simulink library "halin"  (R2021b)
settings: Solver=VariableStepAuto  StartTime=0.0  StopTime=10.0  RelTol=1e-3
undefined symbols (not defined in the file): KHAL_CAN1ABM1E2E_flg, KHAL_CAN1ESC1E2E_flg, KHAL_CAN1ESC5E2E_flg, KHAL_CAN1ESC7E2E_flg, KHAL_CAN1FCM2E2E_flg, KHAL_CAN1FCM3E2E_flg, KHAL_CAN1FCM4E2E_flg, KHAL_CAN3BMS1E2E_flg, KHAL_CAN3BMS6E2E_flg, KHAL_CAN3CCU1E2E_flg, KHAL_CAN3CCU2E2E_flg, KHAL_CAN3MCUF1E2E_flg, KHAL_CAN3MCUR1E2E_flg, KHAL_CAN3Shifter1E2E_flg, TRUE
libraries: simulink x420, FVT_lib x149, hcu_lib x49
(part 2 of 14)

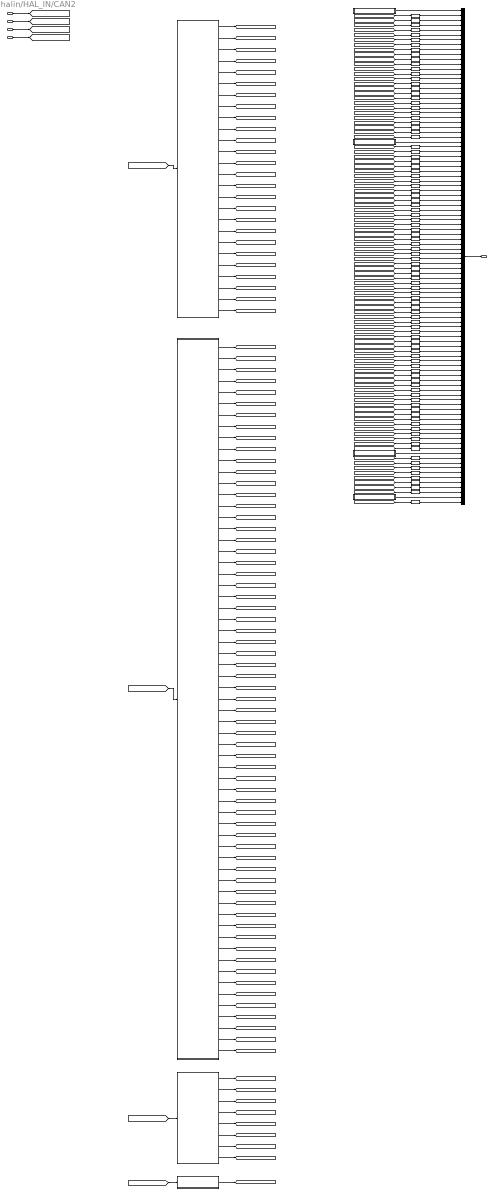
== system halin/HAL_IN/CAN2 ==
  DT_CAN2_SG_IVI1 : Inport
  DT_CAN2_SG_IVI2 : Inport  Port=2
  DT_CAN2_SG_IVI6 : Inport  Port=3
  DT_CAN2_SG_METER1 : Inport  Port=4
  IVI1 : Subsystem
  IVI2 : Subsystem
  IVI6 : Subsystem
  METER1 : Subsystem
  UnitConverter{,1,11,25,28..30,32,37..39,43..44,46,48..50,52..53,57,66..68,70,75,77,80,82,89..90} (30 alike) : DataTypeConversion  OutDataTypeStr=uint8
  UnitConverter{2,4..8,10,12..24,26..27,31,33..36,40,45,47,51,54..56,58..60,69,71,73..74,76,78..79,81,83..86} (49 alike) : DataTypeConversion  OutDataTypeStr=boolean
  UnitConverter{3,9,41,61..65,72,87..88,91..97} (18 alike) : DataTypeConversion  OutDataTypeStr=single
  UnitConverter42 : DataTypeConversion  OutDataTypeStr=uint32
  VHAL_CANMsgInvalidIVI1_flg : Subsystem  AncestorBlock=FVT_lib/hal/MsgTimeoutJudge_CAN_AUTOSAR
      mask help: MeasumentTrigerEvent
      mask Display: fprintf('MsgTimeoutJudge_CAN\nAUTOSAR');
  VHAL_CANMsgInvalidIVI2_flg : Subsystem  AncestorBlock=FVT_lib/hal/MsgTimeoutJudge_CAN_AUTOSAR
      mask help: MeasumentTrigerEvent
      mask Display: fprintf('MsgTimeoutJudge_CAN\nAUTOSAR');
  VHAL_CANMsgInvalidIVI6_flg : Subsystem  AncestorBlock=FVT_lib/hal/MsgTimeoutJudge_CAN_AUTOSAR
      mask help: MeasumentTrigerEvent
      mask Display: fprintf('MsgTimeoutJudge_CAN\nAUTOSAR');
  VHAL_CANMsgInvalidMETER1_flg : Subsystem  AncestorBlock=FVT_lib/hal/MsgTimeoutJudge_CAN_AUTOSAR
      mask help: MeasumentTrigerEvent
      mask Display: fprintf('MsgTimeoutJudge_CAN\nAUTOSAR');
  bus_creator : BusCreator  Inputs=102
  HAL_CAN2_outputs : Outport
  wires:
  DT_CAN2_SG_IVI1/1 -> [DT_CAN2_SG_IVI1]
  DT_CAN2_SG_IVI2/1 -> [DT_CAN2_SG_IVI2]
  DT_CAN2_SG_IVI6/1 -> [DT_CAN2_SG_IVI6]
  DT_CAN2_SG_METER1/1 -> [DT_CAN2_SG_METER1]
  [DT_CAN2_SG_IVI1] -> IVI1/1(DT_CAN2_SG_IVI1)
  [DT_CAN2_SG_IVI2] -> IVI2/1(DT_CAN2_SG_IVI2)
  [DT_CAN2_SG_IVI6] -> IVI6/1(DT_CAN2_SG_IVI6)
  [DT_CAN2_SG_METER1] -> METER1/1(DT_CAN2_SG_METER1)
  bus_creator/1 -> HAL_CAN2_outputs/1
  VHAL_CANMsgInvalidIVI1_flg/1(Out) -> bus_creator/1
  IVI1/1(VHAL_AmbLightColorSet_enum) -> [VHAL_AmbLightColorSet_enum]
  UnitConverter/1 -> bus_creator/2  "VHAL_AmbLightColorSet_enum"
  [VHAL_AmbLightColorSet_enum] -> UnitConverter/1
  IVI1/2(VHAL_AmbLightUserSet_enum) -> [VHAL_AmbLightUserSet_enum]
  UnitConverter1/1 -> bus_creator/3  "VHAL_AmbLightUserSet_enum"
  [VHAL_AmbLightUserSet_enum] -> UnitConverter1/1
  IVI1/3(VHAL_BrkAbnGoReadySW_flg) -> [VHAL_BrkAbnGoReadySW_flg]
  UnitConverter2/1 -> bus_creator/4  "VHAL_BrkAbnGoReadySW_flg"
  [VHAL_BrkAbnGoReadySW_flg] -> UnitConverter2/1
  IVI1/4(VHAL_DRAmbLightBrightnessSet_pct) -> [VHAL_DRAmbLightBrightnessSet_pct]
  UnitConverter3/1 -> bus_creator/5  "VHAL_DRAmbLightBrightnessSet_pct"
  [VHAL_DRAmbLightBrightnessSet_pct] -> UnitConverter3/1
  IVI1/5(VHAL_FCPFrEvtBtnACMaxReq_flg) -> [VHAL_FCPFrEvtBtnACMaxReq_flg]
  UnitConverter4/1 -> bus_creator/6  "VHAL_FCPFrEvtBtnACMaxReq_flg"
  [VHAL_FCPFrEvtBtnACMaxReq_flg] -> UnitConverter4/1
  IVI1/6(VHAL_FCPFrEvtBtnACReq_flg) -> [VHAL_FCPFrEvtBtnACReq_flg]
  UnitConverter5/1 -> bus_creator/7  "VHAL_FCPFrEvtBtnACReq_flg"
  [VHAL_FCPFrEvtBtnACReq_flg] -> UnitConverter5/1
  IVI1/7(VHAL_FCPFrEvtBtnAutoReq_flg) -> [VHAL_FCPFrEvtBtnAutoReq_flg]
  UnitConverter6/1 -> bus_creator/8  "VHAL_FCPFrEvtBtnAutoReq_flg"
  [VHAL_FCPFrEvtBtnAutoReq_flg] -> UnitConverter6/1
  IVI1/8(VHAL_FCPFrEvtBtnSyncReq_flg) -> [VHAL_FCPFrEvtBtnSyncReq_flg]
  UnitConverter7/1 -> bus_creator/9  "VHAL_FCPFrEvtBtnSyncReq_flg"
  [VHAL_FCPFrEvtBtnSyncReq_flg] -> UnitConverter7/1
  IVI1/9(VHAL_FCPMidEvtBtnAutoReq_flg) -> [VHAL_FCPMidEvtBtnAutoReq_flg]
  UnitConverter8/1 -> bus_creator/10  "VHAL_FCPMidEvtBtnAutoReq_flg"
  [VHAL_FCPMidEvtBtnAutoReq_flg] -> UnitConverter8/1
  IVI1/10(VHAL_IPAmbLightBrightnessSet_pct) -> [VHAL_IPAmbLightBrightnessSet_pct]
  UnitConverter9/1 -> bus_creator/11  "VHAL_IPAmbLightBrightnessSet_pct"
  [VHAL_IPAmbLightBrightnessSet_pct] -> UnitConverter9/1
  IVI1/11(VHAL_IVILockSoundSWSta_flg) -> [VHAL_IVILockSoundSWSta_flg]
  UnitConverter10/1 -> bus_creator/12  "VHAL_IVILockSoundSWSta_flg"
  [VHAL_IVILockSoundSWSta_flg] -> UnitConverter10/1
  IVI1/12(VHAL_IVIOTAUpdSta_enum) -> [VHAL_IVIOTAUpdSta_enum]
  UnitConverter11/1 -> bus_creator/13  "VHAL_IVIOTAUpdSta_enum"
  [VHAL_IVIOTAUpdSta_enum] -> UnitConverter11/1
  IVI1/13(VHAL_LINKtoDrive_flg) -> [VHAL_LINKtoDrive_flg]
  UnitConverter12/1 -> bus_creator/14  "VHAL_LINKtoDrive_flg"
  [VHAL_LINKtoDrive_flg] -> UnitConverter12/1
  IVI1/14(VHAL_OTACancelDLReq_flg) -> [VHAL_OTACancelDLReq_flg]
  UnitConverter13/1 -> bus_creator/15  "VHAL_OTACancelDLReq_flg"
  [VHAL_OTACancelDLReq_flg] -> UnitConverter13/1
  IVI1/15(VHAL_OTACompNTFYPres_flg) -> [VHAL_OTACompNTFYPres_flg]
  UnitConverter14/1 -> bus_creator/16  "VHAL_OTACompNTFYPres_flg"
  [VHAL_OTACompNTFYPres_flg] -> UnitConverter14/1
  IVI1/16(VHAL_OTADLReq_flg) -> [VHAL_OTADLReq_flg]
  UnitConverter15/1 -> bus_creator/17  "VHAL_OTADLReq_flg"
  [VHAL_OTADLReq_flg] -> UnitConverter15/1
  IVI1/17(VHAL_OTASuspendDLReq_flg) -> [VHAL_OTASuspendDLReq_flg]
  UnitConverter16/1 -> bus_creator/18  "VHAL_OTASuspendDLReq_flg"
  [VHAL_OTASuspendDLReq_flg] -> UnitConverter16/1
  IVI1/18(VHAL_OTAUpdStartReq_flg) -> [VHAL_OTAUpdStartReq_flg]
  UnitConverter17/1 -> bus_creator/19  "VHAL_OTAUpdStartReq_flg"
  [VHAL_OTAUpdStartReq_flg] -> UnitConverter17/1
  IVI1/19(VHAL_OpenDrOpenWdoSW_flg) -> [VHAL_OpenDrOpenWdoSW_flg]
  UnitConverter18/1 -> bus_creator/20  "VHAL_OpenDrOpenWdoSW_flg"
  [VHAL_OpenDrOpenWdoSW_flg] -> UnitConverter18/1
  IVI1/20(VHAL_PWCLOSEIMD_flg) -> [VHAL_PWCLOSEIMD_flg]
  UnitConverter19/1 -> bus_creator/21  "VHAL_PWCLOSEIMD_flg"
  [VHAL_PWCLOSEIMD_flg] -> UnitConverter19/1
  IVI1/21(VHAL_PWCONTINUEUSE_flg) -> [VHAL_PWCONTINUEUSE_flg]
  UnitConverter20/1 -> bus_creator/22  "VHAL_PWCONTINUEUSE_flg"
  [VHAL_PWCONTINUEUSE_flg] -> UnitConverter20/1
  IVI1/22(VHAL_SchedOTAwake_flg) -> [VHAL_SchedOTAwake_flg]
  UnitConverter21/1 -> bus_creator/23  "VHAL_SchedOTAwake_flg"
  [VHAL_SchedOTAwake_flg] -> UnitConverter21/1
  IVI1/23(VHAL_SmartEcoModeSW_flg) -> [VHAL_SmartEcoModeSW_flg]
  UnitConverter22/1 -> bus_creator/24  "VHAL_SmartEcoModeSW_flg"
  [VHAL_SmartEcoModeSW_flg] -> UnitConverter22/1
  IVI1/24(VHAL_UpdCountdownCancel_flg) -> [VHAL_UpdCountdownCancel_flg]
  UnitConverter23/1 -> bus_creator/25  "VHAL_UpdCountdownCancel_flg"
  [VHAL_UpdCountdownCancel_flg] -> UnitConverter23/1
  IVI1/25(VHAL_UpdCountdownSkip_flg) -> [VHAL_UpdCountdownSkip_flg]
  UnitConverter24/1 -> bus_creator/26  "VHAL_UpdCountdownSkip_flg"
  [VHAL_UpdCountdownSkip_flg] -> UnitConverter24/1
  IVI1/26(VHAL_VehACModReq_enum) -> [VHAL_VehACModReq_enum]
  UnitConverter25/1 -> bus_creator/27  "VHAL_VehACModReq_enum"
  [VHAL_VehACModReq_enum] -> UnitConverter25/1
  VHAL_CANMsgInvalidIVI2_flg/1(Out) -> bus_creator/28
  IVI2/1(VHAL_AVMErrSTA_flg) -> [VHAL_AVMErrSTA_flg]
  UnitConverter26/1 -> bus_creator/29  "VHAL_AVMErrSTA_flg"
  [VHAL_AVMErrSTA_flg] -> UnitConverter26/1
  IVI2/2(VHAL_AVMOFFRecButt_flg) -> [VHAL_AVMOFFRecButt_flg]
  UnitConverter27/1 -> bus_creator/30  "VHAL_AVMOFFRecButt_flg"
  [VHAL_AVMOFFRecButt_flg] -> UnitConverter27/1
  IVI2/3(VHAL_AVMParkingmode_enum) -> [VHAL_AVMParkingmode_enum]
  UnitConverter28/1 -> bus_creator/31  "VHAL_AVMParkingmode_enum"
  [VHAL_AVMParkingmode_enum] -> UnitConverter28/1
  IVI2/4(VHAL_AVMparkingcancel_enum) -> [VHAL_AVMparkingcancel_enum]
  UnitConverter29/1 -> bus_creator/32  "VHAL_AVMparkingcancel_enum"
  [VHAL_AVMparkingcancel_enum] -> UnitConverter29/1
  IVI2/5(VHAL_AVMparkingexcute_enum) -> [VHAL_AVMparkingexcute_enum]
  UnitConverter30/1 -> bus_creator/33  "VHAL_AVMparkingexcute_enum"
  [VHAL_AVMparkingexcute_enum] -> UnitConverter30/1
  IVI2/6(VHAL_ApproachUnlockSW_flg) -> [VHAL_ApproachUnlockSW_flg]
  UnitConverter31/1 -> bus_creator/34  "VHAL_ApproachUnlockSW_flg"
  [VHAL_ApproachUnlockSW_flg] -> UnitConverter31/1
  IVI2/7(VHAL_CAASSw_enum) -> [VHAL_CAASSw_enum]
  UnitConverter32/1 -> bus_creator/35  "VHAL_CAASSw_enum"
  [VHAL_CAASSw_enum] -> UnitConverter32/1
  IVI2/8(VHAL_CDLLockButt_flg) -> [VHAL_CDLLockButt_flg]
  UnitConverter33/1 -> bus_creator/36  "VHAL_CDLLockButt_flg"
  [VHAL_CDLLockButt_flg] -> UnitConverter33/1
  IVI2/9(VHAL_CDLUnlockButt_flg) -> [VHAL_CDLUnlockButt_flg]
  UnitConverter34/1 -> bus_creator/37  "VHAL_CDLUnlockButt_flg"
  [VHAL_CDLUnlockButt_flg] -> UnitConverter34/1
  IVI2/10(VHAL_DSEATantiset_flg) -> [VHAL_DSEATantiset_flg]
  UnitConverter35/1 -> bus_creator/38  "VHAL_DSEATantiset_flg"
  [VHAL_DSEATantiset_flg] -> UnitConverter35/1
  IVI2/11(VHAL_DSEATentryfunset_flg) -> [VHAL_DSEATentryfunset_flg]
  UnitConverter36/1 -> bus_creator/39  "VHAL_DSEATentryfunset_flg"
  [VHAL_DSEATentryfunset_flg] -> UnitConverter36/1
  IVI2/12(VHAL_DSEATventreq_enum) -> [VHAL_DSEATventreq_enum]
  UnitConverter37/1 -> bus_creator/40  "VHAL_DSEATventreq_enum"
  [VHAL_DSEATventreq_enum] -> UnitConverter37/1
  IVI2/13(VHAL_ESCSWCmd_enum) -> [VHAL_ESCSWCmd_enum]
  UnitConverter38/1 -> bus_creator/41  "VHAL_ESCSWCmd_enum"
  [VHAL_ESCSWCmd_enum] -> UnitConverter38/1
  IVI2/14(VHAL_FSOffSw_enum) -> [VHAL_FSOffSw_enum]
  UnitConverter39/1 -> bus_creator/42  "VHAL_FSOffSw_enum"
  [VHAL_FSOffSw_enum] -> UnitConverter39/1
  IVI2/15(VHAL_FollowMeSW_flg) -> [VHAL_FollowMeSW_flg]
  UnitConverter40/1 -> bus_creator/43  "VHAL_FollowMeSW_flg"
  [VHAL_FollowMeSW_flg] -> UnitConverter40/1
  IVI2/16(VHAL_GPSLAT_s) -> [VHAL_GPSLAT_s]
  UnitConverter41/1 -> bus_creator/44  "VHAL_GPSLAT_s"
  [VHAL_GPSLAT_s] -> UnitConverter41/1
  IVI2/17(VHAL_GPSLONG_enum) -> [VHAL_GPSLONG_enum]
  UnitConverter42/1 -> bus_creator/45  "VHAL_GPSLONG_enum"
  [VHAL_GPSLONG_enum] -> UnitConverter42/1
  IVI2/18(VHAL_HeadLampSW_enum) -> [VHAL_HeadLampSW_enum]
  UnitConverter43/1 -> bus_creator/46  "VHAL_HeadLampSW_enum"
  [VHAL_HeadLampSW_enum] -> UnitConverter43/1
  IVI2/19(VHAL_HoodLatchSW_enum) -> [VHAL_HoodLatchSW_enum]
  UnitConverter44/1 -> bus_creator/47  "VHAL_HoodLatchSW_enum"
  [VHAL_HoodLatchSW_enum] -> UnitConverter44/1
  IVI2/20(VHAL_IVICreepSWReq_flg) -> [VHAL_IVICreepSWReq_flg]
  UnitConverter45/1 -> bus_creator/48  "VHAL_IVICreepSWReq_flg"
  [VHAL_IVICreepSWReq_flg] -> UnitConverter45/1
  IVI2/21(VHAL_IVIISAOffsetSpd_enum) -> [VHAL_IVIISAOffsetSpd_enum]
  UnitConverter46/1 -> bus_creator/49  "VHAL_IVIISAOffsetSpd_enum"
  [VHAL_IVIISAOffsetSpd_enum] -> UnitConverter46/1
  IVI2/22(VHAL_IVINightModeSta_flg) -> [VHAL_IVINightModeSta_flg]
  UnitConverter47/1 -> bus_creator/50  "VHAL_IVINightModeSta_flg"
  [VHAL_IVINightModeSta_flg] -> UnitConverter47/1
  IVI2/23(VHAL_IVIPTGModeSW_enum) -> [VHAL_IVIPTGModeSW_enum]
  UnitConverter48/1 -> bus_creator/51  "VHAL_IVIPTGModeSW_enum"
  [VHAL_IVIPTGModeSW_enum] -> UnitConverter48/1
  IVI2/24(VHAL_IVIPTGOpenHeight_enum) -> [VHAL_IVIPTGOpenHeight_enum]
  UnitConverter49/1 -> bus_creator/52  "VHAL_IVIPTGOpenHeight_enum"
  [VHAL_IVIPTGOpenHeight_enum] -> UnitConverter49/1
  IVI2/25(VHAL_IVIPTGStaSW_enum) -> [VHAL_IVIPTGStaSW_enum]
  UnitConverter50/1 -> bus_creator/53  "VHAL_IVIPTGStaSW_enum"
  [VHAL_IVIPTGStaSW_enum] -> UnitConverter50/1
  IVI2/26(VHAL_IVIPTGUSStaSW_flg) -> [VHAL_IVIPTGUSStaSW_flg]
  UnitConverter51/1 -> bus_creator/54  "VHAL_IVIPTGUSStaSW_flg"
  [VHAL_IVIPTGUSStaSW_flg] -> UnitConverter51/1
  IVI2/27(VHAL_IVIPWModeReq_enum) -> [VHAL_IVIPWModeReq_enum]
  UnitConverter52/1 -> bus_creator/55  "VHAL_IVIPWModeReq_enum"
  [VHAL_IVIPWModeReq_enum] -> UnitConverter52/1
  IVI2/28(VHAL_IVIPwrLockSW_enum) -> [VHAL_IVIPwrLockSW_enum]
  UnitConverter53/1 -> bus_creator/56  "VHAL_IVIPwrLockSW_enum"
  [VHAL_IVIPwrLockSW_enum] -> UnitConverter53/1
  IVI2/29(VHAL_IVIPwroffreq_flg) -> [VHAL_IVIPwroffreq_flg]
  UnitConverter54/1 -> bus_creator/57  "VHAL_IVIPwroffreq_flg"
  [VHAL_IVIPwroffreq_flg] -> UnitConverter54/1
  IVI2/30(VHAL_IVIRRDefReq_flg) -> [VHAL_IVIRRDefReq_flg]
  UnitConverter55/1 -> bus_creator/58  "VHAL_IVIRRDefReq_flg"
  [VHAL_IVIRRDefReq_flg] -> UnitConverter55/1
  IVI2/31(VHAL_IVIReqV2L_flg) -> [VHAL_IVIReqV2L_flg]
  UnitConverter56/1 -> bus_creator/59  "VHAL_IVIReqV2L_flg"
  [VHAL_IVIReqV2L_flg] -> UnitConverter56/1
  IVI2/32(VHAL_IVIScreen_enum) -> [VHAL_IVIScreen_enum]
  UnitConverter57/1 -> bus_creator/60  "VHAL_IVIScreen_enum"
  [VHAL_IVIScreen_enum] -> UnitConverter57/1
  IVI2/33(VHAL_IVIStatus_flg) -> [VHAL_IVIStatus_flg]
  UnitConverter58/1 -> bus_creator/61  "VHAL_IVIStatus_flg"
  [VHAL_IVIStatus_flg] -> UnitConverter58/1
  IVI2/34(VHAL_IVITriggerreq_flg) -> [VHAL_IVITriggerreq_flg]
  UnitConverter59/1 -> bus_creator/62  "VHAL_IVITriggerreq_flg"
  [VHAL_IVITriggerreq_flg] -> UnitConverter59/1
  IVI2/35(VHAL_IVIWIMAINSW_flg) -> [VHAL_IVIWIMAINSW_flg]
  UnitConverter60/1 -> bus_creator/63  "VHAL_IVIWIMAINSW_flg"
  [VHAL_IVIWIMAINSW_flg] -> UnitConverter60/1
  IVI2/36(VHAL_LDrvControlCommand_pct) -> [VHAL_LDrvControlCommand_pct]
  UnitConverter61/1 -> bus_creator/64  "VHAL_LDrvControlCommand_pct"
  [VHAL_LDrvControlCommand_pct] -> UnitConverter61/1
  IVI2/37(VHAL_LPasControlCommand_pct) -> [VHAL_LPasControlCommand_pct]
  UnitConverter62/1 -> bus_creator/65  "VHAL_LPasControlCommand_pct"
  [VHAL_LPasControlCommand_pct] -> UnitConverter62/1
  IVI2/38(VHAL_LRLDControlCommand_pct) -> [VHAL_LRLDControlCommand_pct]
  UnitConverter63/1 -> bus_creator/66  "VHAL_LRLDControlCommand_pct"
  [VHAL_LRLDControlCommand_pct] -> UnitConverter63/1
  IVI2/39(VHAL_LRRDControlCommand_pct) -> [VHAL_LRRDControlCommand_pct]
  UnitConverter64/1 -> bus_creator/67  "VHAL_LRRDControlCommand_pct"
  [VHAL_LRRDControlCommand_pct] -> UnitConverter64/1
  IVI2/40(VHAL_MFRDNBrightReq_pct) -> [VHAL_MFRDNBrightReq_pct]
  UnitConverter65/1 -> bus_creator/68  "VHAL_MFRDNBrightReq_pct"
  [VHAL_MFRDNBrightReq_pct] -> UnitConverter65/1
  IVI2/41(VHAL_OFFACMODE_enum) -> [VHAL_OFFACMODE_enum]
  UnitConverter66/1 -> bus_creator/69  "VHAL_OFFACMODE_enum"
  [VHAL_OFFACMODE_enum] -> UnitConverter66/1
  IVI2/42(VHAL_PSEATventreq_enum) -> [VHAL_PSEATventreq_enum]
  UnitConverter67/1 -> bus_creator/70  "VHAL_PSEATventreq_enum"
  [VHAL_PSEATventreq_enum] -> UnitConverter67/1
  IVI2/43(VHAL_PerdV2L_enum) -> [VHAL_PerdV2L_enum]
  UnitConverter68/1 -> bus_creator/71  "VHAL_PerdV2L_enum"
  [VHAL_PerdV2L_enum] -> UnitConverter68/1
  IVI2/44(VHAL_RFogLampSW_flg) -> [VHAL_RFogLampSW_flg]
  UnitConverter69/1 -> bus_creator/72  "VHAL_RFogLampSW_flg"
  [VHAL_RFogLampSW_flg] -> UnitConverter69/1
  IVI2/45(VHAL_RollModeSWCmd_enum) -> [VHAL_RollModeSWCmd_enum]
  UnitConverter70/1 -> bus_creator/73  "VHAL_RollModeSWCmd_enum"
  [VHAL_RollModeSWCmd_enum] -> UnitConverter70/1
  IVI2/46(VHAL_RoomLampMode_flg) -> [VHAL_RoomLampMode_flg]
  UnitConverter71/1 -> bus_creator/74  "VHAL_RoomLampMode_flg"
  [VHAL_RoomLampMode_flg] -> UnitConverter71/1
  IVI2/47(VHAL_SOCV2LLimit_pct) -> [VHAL_SOCV2LLimit_pct]
  UnitConverter72/1 -> bus_creator/75  "VHAL_SOCV2LLimit_pct"
  [VHAL_SOCV2LLimit_pct] -> UnitConverter72/1
  IVI2/48(VHAL_SchedChgbutt_flg) -> [VHAL_SchedChgbutt_flg]
  UnitConverter73/1 -> bus_creator/76  "VHAL_SchedChgbutt_flg"
  [VHAL_SchedChgbutt_flg] -> UnitConverter73/1
  IVI2/49(VHAL_SchedChgwake_flg) -> [VHAL_SchedChgwake_flg]
  UnitConverter74/1 -> bus_creator/77  "VHAL_SchedChgwake_flg"
  [VHAL_SchedChgwake_flg] -> UnitConverter74/1
  IVI2/50(VHAL_SenstivityPosition_enum) -> [VHAL_SenstivityPosition_enum]
  UnitConverter75/1 -> bus_creator/78  "VHAL_SenstivityPosition_enum"
  [VHAL_SenstivityPosition_enum] -> UnitConverter75/1
  IVI2/51(VHAL_SetUnlockSingle_flg) -> [VHAL_SetUnlockSingle_flg]
  UnitConverter76/1 -> bus_creator/79  "VHAL_SetUnlockSingle_flg"
  [VHAL_SetUnlockSingle_flg] -> UnitConverter76/1
  IVI2/52(VHAL_TCSSWCmd_enum) -> [VHAL_TCSSWCmd_enum]
  UnitConverter77/1 -> bus_creator/80  "VHAL_TCSSWCmd_enum"
  [VHAL_TCSSWCmd_enum] -> UnitConverter77/1
  IVI2/53(VHAL_TPMSCaliButt_flg) -> [VHAL_TPMSCaliButt_flg]
  UnitConverter78/1 -> bus_creator/81  "VHAL_TPMSCaliButt_flg"
  [VHAL_TPMSCaliButt_flg] -> UnitConverter78/1
  IVI2/54(VHAL_TPMSResButt_flg) -> [VHAL_TPMSResButt_flg]
  UnitConverter79/1 -> bus_creator/82  "VHAL_TPMSResButt_flg"
  [VHAL_TPMSResButt_flg] -> UnitConverter79/1
  IVI2/55(VHAL_TurnSwTimeSet_enum) -> [VHAL_TurnSwTimeSet_enum]
  UnitConverter80/1 -> bus_creator/83  "VHAL_TurnSwTimeSet_enum"
  [VHAL_TurnSwTimeSet_enum] -> UnitConverter80/1
  IVI2/56(VHAL_WalkawayLockSW_flg) -> [VHAL_WalkawayLockSW_flg]
  UnitConverter81/1 -> bus_creator/84  "VHAL_WalkawayLockSW_flg"
  [VHAL_WalkawayLockSW_flg] -> UnitConverter81/1
  IVI2/57(VHAL_sigAirIntenZon1Req_enum) -> [VHAL_sigAirIntenZon1Req_enum]
  UnitConverter82/1 -> bus_creator/85  "VHAL_sigAirIntenZon1Req_enum"
  [VHAL_sigAirIntenZon1Req_enum] -> UnitConverter82/1
  IVI2/58(VHAL_sigDfrstReq_flg) -> [VHAL_sigDfrstReq_flg]
  UnitConverter83/1 -> bus_creator/86  "VHAL_sigDfrstReq_flg"
  [VHAL_sigDfrstReq_flg] -> UnitConverter83/1
  IVI2/59(VHAL_sigFaceReq_flg) -> [VHAL_sigFaceReq_flg]
  UnitConverter84/1 -> bus_creator/87  "VHAL_sigFaceReq_flg"
  [VHAL_sigFaceReq_flg] -> UnitConverter84/1
  IVI2/60(VHAL_sigFootReq_flg) -> [VHAL_sigFootReq_flg]
  UnitConverter85/1 -> bus_creator/88  "VHAL_sigFootReq_flg"
  [VHAL_sigFootReq_flg] -> UnitConverter85/1
  IVI2/61(VHAL_sigRecircReq_flg) -> [VHAL_sigRecircReq_flg]
  UnitConverter86/1 -> bus_creator/89  "VHAL_sigRecircReq_flg"
  [VHAL_sigRecircReq_flg] -> UnitConverter86/1
  IVI2/62(VHAL_sigSetTempZon1Req_C) -> [VHAL_sigSetTempZon1Req_C]
  UnitConverter87/1 -> bus_creator/90  "VHAL_sigSetTempZon1Req_C"
  [VHAL_sigSetTempZon1Req_C] -> UnitConverter87/1
  IVI2/63(VHAL_sigSetTempZon2Req_C) -> [VHAL_sigSetTempZon2Req_C]
  UnitConverter88/1 -> bus_creator/91  "VHAL_sigSetTempZon2Req_C"
  [VHAL_sigSetTempZon2Req_C] -> UnitConverter88/1
  VHAL_CANMsgInvalidIVI6_flg/1(Out) -> bus_creator/92
  IVI6/1(VHAL_IVILocatedSTA_enum) -> [VHAL_IVILocatedSTA_enum]
  UnitConverter89/1 -> bus_creator/93  "VHAL_IVILocatedSTA_enum"
  [VHAL_IVILocatedSTA_enum] -> UnitConverter89/1
  IVI6/2(VHAL_IVITimeCheck_enum) -> [VHAL_IVITimeCheck_enum]
  UnitConverter90/1 -> bus_creator/94  "VHAL_IVITimeCheck_enum"
  [VHAL_IVITimeCheck_enum] -> UnitConverter90/1
  IVI6/3(VHAL_IVITimeDay_DAY) -> [VHAL_IVITimeDay_DAY]
  UnitConverter91/1 -> bus_creator/95  "VHAL_IVITimeDay_DAY"
  [VHAL_IVITimeDay_DAY] -> UnitConverter91/1
  IVI6/4(VHAL_IVITimeHour_hr) -> [VHAL_IVITimeHour_hr]
  UnitConverter92/1 -> bus_creator/96  "VHAL_IVITimeHour_hr"
  [VHAL_IVITimeHour_hr] -> UnitConverter92/1
  IVI6/5(VHAL_IVITimeMinute_min) -> [VHAL_IVITimeMinute_min]
  UnitConverter93/1 -> bus_creator/97  "VHAL_IVITimeMinute_min"
  [VHAL_IVITimeMinute_min] -> UnitConverter93/1
  IVI6/6(VHAL_IVITimeMonth_MONTH) -> [VHAL_IVITimeMonth_MONTH]
  UnitConverter94/1 -> bus_creator/98  "VHAL_IVITimeMonth_MONTH"
  [VHAL_IVITimeMonth_MONTH] -> UnitConverter94/1
  IVI6/7(VHAL_IVITimeSecond_s) -> [VHAL_IVITimeSecond_s]
  UnitConverter95/1 -> bus_creator/99  "VHAL_IVITimeSecond_s"
  [VHAL_IVITimeSecond_s] -> UnitConverter95/1
  IVI6/8(VHAL_IVITimeYear_YEAR) -> [VHAL_IVITimeYear_YEAR]
  UnitConverter96/1 -> bus_creator/100  "VHAL_IVITimeYear_YEAR"
  [VHAL_IVITimeYear_YEAR] -> UnitConverter96/1
  VHAL_CANMsgInvalidMETER1_flg/1(Out) -> bus_creator/101
  METER1/1(VHAL_METERKPHCalcu_kph) -> [VHAL_METERKPHCalcu_kph]
  UnitConverter97/1 -> bus_creator/102  "VHAL_METERKPHCalcu_kph"
  [VHAL_METERKPHCalcu_kph] -> UnitConverter97/1
